simulink model "Nils_Bestehorn_mdl"  (R2021b)
settings: Solver=FixedStepAuto  StartTime=0.0  StopTime=3  FixedStep=0.005  RelTol=1e-3
values from neighbouring files (symbols this model uses):
  alpha = 15*pi/180    (= 0.261799387799)    [Nils_Bestehorn_mfile.m]
  calp = 20000    [Nils_Bestehorn_mfile.m]
  cE = 56115    [Nils_Bestehorn_mfile.m]
  cR = 128000    [Nils_Bestehorn_mfile.m]
  cy = 70000    [Nils_Bestehorn_mfile.m]
  dE = 3195    [Nils_Bestehorn_mfile.m]
  H = 0.15    [Nils_Bestehorn_mfile.m]
  lE = 0.42    [Nils_Bestehorn_mfile.m]
  lR = 0.7    [Nils_Bestehorn_mfile.m]
  mA = 229    [Nils_Bestehorn_mfile.m]
  mR = 31    [Nils_Bestehorn_mfile.m]
  r = 300*10^(-3)    (= 0.3)    [Nils_Bestehorn_mfile.m]
  v = 10    [Nils_Bestehorn_mfile.m]
undefined symbols (not defined in the file or in its folder): sigbuilder_block
libraries: simulink x1
settings Model: Creator=nilsb  LastModifiedBy=nilsb

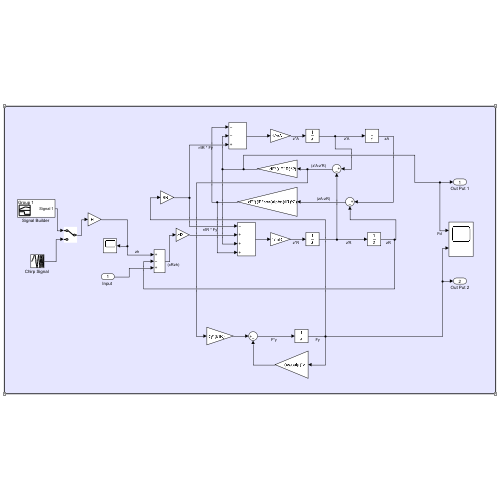
[thumbnail: Simulink's stored preview of the top-level diagram]
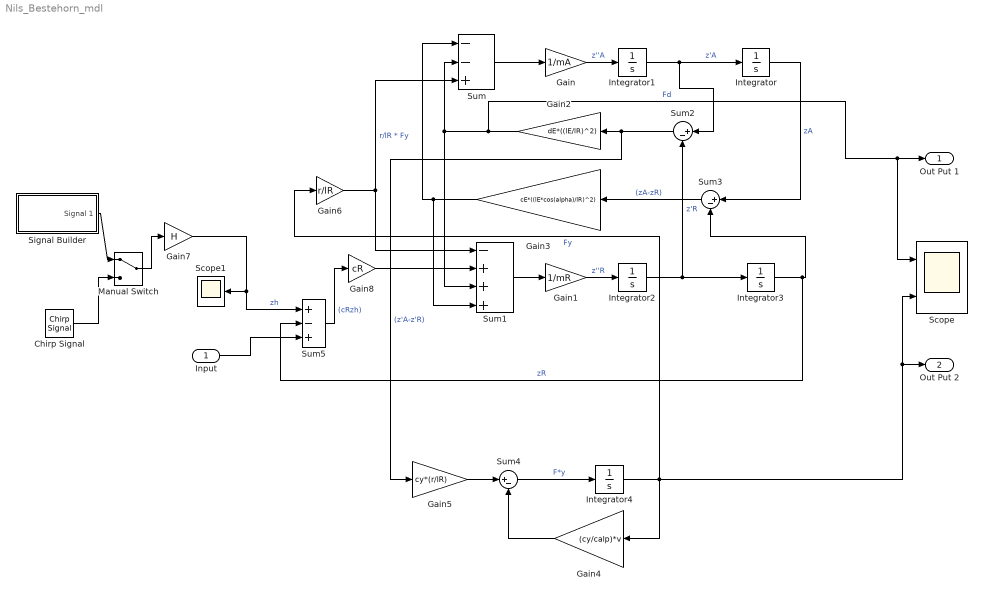
== system Nils_Bestehorn_mdl ==
  "Input " : Inport
  "Chirp Signal " : simulink/Sources/Chirp Signal  f1=0.01  T=20  f2=20
  Gain : Gain  Gain=1/mA
  Gain1 : Gain  Gain=1/mR
  Gain2 : Gain  Gain=dE*((lE/lR)^2)
  Gain3 : Gain  Gain=cE*((lE*cos(alpha)/lR)^2)
  Gain4 : Gain  Gain=(cy/calp)*v
  Gain5 : Gain  Gain=cy*(r/lR)
  Gain6 : Gain  Gain=r/lR
  Gain7 : Gain  Gain=H
  Gain8 : Gain  Gain=cR
  Integrator{,1..4} (5 alike) : Integrator
  Manual Switch : ManualSwitch
  Scope : Scope  NumInputPorts=2
  Scope1 : Scope
  "Signal Builder " : Subsystem  Tag=STV Subsys  LoadFcn=sigbuilder_block('load');  StartFcn=sigbuilder_block('start');  StopFcn=sigbuilder_block('stop');  ClipboardFcn=sigbuilder_block('clipboard');  mask(Sigbuilder block){tuvar=[0:10]}
      mask help: Simulink:masks:SigbuilderBlock_MD
      mask init:
      | if ~strcmp(get_param(bdroot(gcbh),'SimulationStatus'),'stopped') tuvar = sigbuilder_block('maskInit'); end
      settings: CopyFcn=sigbuilder_block('copy');  DeleteFcn=sigbuilder_block('delete');  ModelCloseFcn=sigbuilder_block('modelClose');  PreSaveFcn=sigbuilder_block('preSave');  PauseFcn=sigbuilder_block('pause');  ContinueFcn=sigbuilder_block('continue');  NameChangeFcn=sigbuilder_block('namechange');  OpenFcn=sigbuilder_block('open',[926.25 246.75 550.5 399.75 ]);  CloseFcn=sigbuilder_block('close');
      mask Display: plot(0, 0, 100, 100,[2, 2, 32, 32, 2], [68, 8, 8, 68, 68],[32, 2], [38, 38], [32, 19, 2],[53, 60, 44], [32, 17, 17, 2],[16, 16, 31, 31]);txt = getActiveGroup(gcbh);text(2, 100, txt,'verticalAlignment', 'top');
  Sum : Sum  Inputs=--+
  Sum1 : Sum  Inputs=-+++
  Sum2 : Sum  Inputs=|+-
  Sum3 : Sum  Inputs=|+-
  Sum4 : Sum  Inputs=|+-
  Sum5 : Sum  Inputs=+-+
  Out Put 1 : Outport
  Out Put 2 : Outport  Port=2
  wires:
  Integrator1/1 -> Sum2/1, Integrator/1  "z'A"
  Gain/1 -> Integrator1/1  "z''A"
  Integrator/1 -> Sum3/1  "zA"
  Integrator2/1 -> Integrator3/1, Sum2/2  "z'R"
  Gain1/1 -> Integrator2/1  "z''R"
  Integrator3/1 -> Sum5/2, Sum3/2  "zR"
  Sum/1 -> Gain/1
  Sum1/1 -> Gain1/1
  Sum2/1 -> Gain5/1, Gain2/1  "(z'A-z'R)"
  Sum3/1 -> Gain3/1  "(zA-zR)"
  Gain3/1 -> Sum/1, Sum1/4
  Gain6/1 -> Sum/3, Sum1/1  "r/lR * Fy"
  Sum4/1 -> Integrator4/1  "F*y"
  Gain4/1 -> Sum4/2
  Gain5/1 -> Sum4/1
  "Signal Builder "/1(Signal 1) -> Manual Switch/1
  Integrator4/1 -> Gain6/1, Out Put 2/1, Scope/2, Gain4/1  "Fy"
  Gain2/1 -> Out Put 1/1, Scope/1, Sum/2, Sum1/3  "Fd"
  Gain7/1 -> Sum5/1, Scope1/1  "zh"
  Sum5/1 -> Gain8/1  "(cRzh)"
  Gain8/1 -> Sum1/2
  "Chirp Signal "/1 -> Manual Switch/2
  Manual Switch/1 -> Gain7/1
  "Input "/1 -> Sum5/3

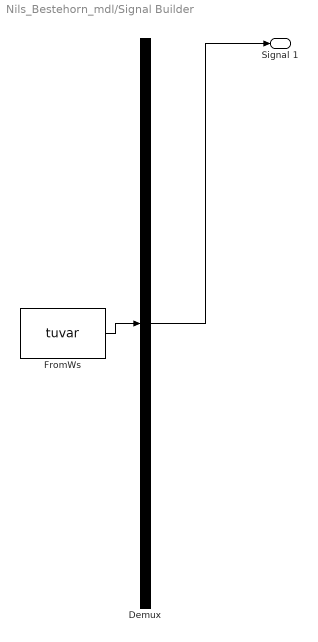
== system Nils_Bestehorn_mdl/Signal Builder  ==
  Demux : Demux  Tag=STV Demux  Outputs=1
      settings: DisplayOption=none
  FromWs : FromWorkspace  Tag=STV FromWs  VariableName=tuvar
      SigBuilderData=|
      | common.afterFinalStr = 'Extrapolate'
      | common.sampleTime = 0
      | dataSet.timeRange = [0 0.5]
      | dataSet.name = 'Group 1'
      | sbobj.Groups.Name = 'Group 1'
      | sbobj.Groups.Signals.Name = 'Signal 1'
      | sbobj.Groups.Signals.XData = [0 0.02 0.1 0.12 0.5]
      | sbobj.Groups.Signals.YData = [0 1 1 0 0]
      | sbobj.Groups.TimeRange = [0 0.5]
  Signal 1 : Outport  Tag=STV Outport
  wires:
  Demux/1 -> Signal 1/1
  FromWs/1 -> Demux/1
